simulink model "model_2"  (R2018b)
settings: Solver=VariableStepAuto  StartTime=0.0  StopTime=1  RelTol=1e-6
undefined symbols (not defined in the file): Angle, Magnitude
libraries: powerlib x7, powerlib_meascontrol x2
CloseFcn:
  | location = 0;
  | fault = 1000;
  | volt_mag = Vm(:,2:4);
  | volt_phase = Vp(:,2:4);
  | curr_mag = Im(:,2:4);
  | curr_phase = Ip(:,2:4);
  | logg = [volt_mag,volt_phase,curr_mag,curr_phase];
  | data = xlsread('fdata');
  | data = [data,logg];
  | xlswrite('fdata',data);
settings Model: Creator=Edagotti Pavankumar  LastModifiedBy=Edagotti Pavankumar
settings SolverCC: ZeroCrossAlgorithm=Adaptive
settings DebuggingCC: IgnoredZcDiagnostic=none

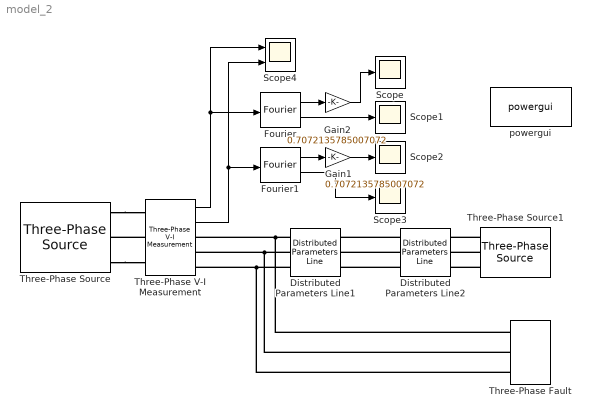
== system model_2 ==
  Distributed Parameters Line1 : powerlib/Elements/Distributed Parameters Line  Phases=3  Frequency=50  Resistance=[0.0238 0.3885]  Inductance="[9.5095e-4  3.25089e-3]"  Capacitance=[12.74e-9 7.751e-9]  Length=180  x1=[8.48515176744739e-11 220461.22116644 220461.22116644;314.159265358979 314.159265358979 314.159265358979;1.82735701330617 0.32640586240689 -1.24439046438801]  x2=[9.7617214960328e-11 220937.914601075 220937.914601075;314.159265358979 314.159265358979 314.159265358979;-2.31830274955501 0.326237122162251 -1.24455920463265]  x3=[1.11025186173268e-12 802.312186393221 802.312186393221;314.159265358979 314.159265358979 314.159265358979;3.10271250295735 0.216627142271568 -1.35416918452333]  x4=[9.65269565360141e-13 802.283126585131 802.283126585132;314.159265358979 314.159265358979 314.159265358979;-0.809925232756074 0.238414402370631 -1.33238192442426]  x5=0.00090355066699992  V1=[8.485e-11 2.205e+05 2.205e+05;314.2 314.2 314.2;1.827 0.3264 -1.244]  V2=[9.762e-11 2.209e+05 2.209e+05;314.2 314.2 314.2;-2.318 0.3262 -1.245]  I1=[1.11e-12 802.3 802.3;314.2 314.2 314.2;3.103 0.2166 -1.354]  I2=[9.653e-13 802.3 802.3;314.2 314.2 314.2;-0.8099 0.2384 -1.332]  nHarmo=1  Measurements=None
      settings: SourceProductName=Simscape Power Systems
  Distributed Parameters Line2 : powerlib/Elements/Distributed Parameters Line  Phases=3  Frequency=50  Resistance=[0.0238 0.3885]  Inductance="[9.5095e-4  3.25089e-3]"  Capacitance=[12.74e-9 7.751e-9]  Length=20  x1=[9.7617214960328e-11 220937.914601075 220937.914601075;314.159265358979 314.159265358979 314.159265358979;-2.06598380399118 0.501194963128134 -1.06960136366676]  x2=[7.31224690470909e-11 220461.378018612 220461.378018612;314.159265358979 314.159265358979 314.159265358979;1.43958780610826 0.50136822766239 -1.06942809913251]  x3=[1.14752079646779e-11 810.765041180401 810.765041180394;314.159265358979 314.159265358979 314.159265358979;-0.0610879160973727 0.588705873026849 -0.982090453768037]  x4=[2.68747980507289e-12 810.674115725578 810.674115725588;314.159265358979 314.159265358979 314.159265358979;-2.96130497430385 0.391966806258209 -1.1788295205367]  x5=0.000100394518555547  V1=[9.762e-11 2.209e+05 2.209e+05;314.2 314.2 314.2;-2.066 0.5012 -1.07]  V2=[7.312e-11 2.205e+05 2.205e+05;314.2 314.2 314.2;1.44 0.5014 -1.069]  I1=[1.148e-11 810.8 810.8;314.2 314.2 314.2;-0.06109 0.5887 -0.9821]  I2=[2.687e-12 810.7 810.7;314.2 314.2 314.2;-2.961 0.392 -1.179]  nHarmo=1  Measurements=None
      settings: SourceProductName=Simscape Power Systems
  Fourier : powerlib_meascontrol/Measurements/Fourier  Freq=50  n=1  InInit=[0, 0]  Ts=0
      settings: SourceProductName=Simscape Power Systems
  Fourier1 : powerlib_meascontrol/Measurements/Fourier  Freq=50  n=1  InInit=[0, 0]  Ts=0
      settings: SourceProductName=Simscape Power Systems
  Gain1 : Gain  Gain=0.7072135785007072
  Gain2 : Gain  Gain=0.7072135785007072
  Scope{,1..3} (4 alike) : Scope
  Scope4 : Scope  NumInputPorts=2
  Three-Phase V-I Measurement : powerlib/Measurements/Three-Phase V-I Measurement  VoltageMeasurement=phase-to-ground  SetLabelV=off  LabelV=Vabc  Vpu=on  VpuLL=off  CurrentMeasurement=yes  SetLabelI=off  LabelI=Iabc  Ipu=on  Pbase=100e6  Vbase=220e3  OutputType=Magnitude-Angle  PhasorSimulation=off  PSBequivalent=0
  Three-Phase Fault : powerlib/Elements/Three-Phase Fault  InitialStates=0  FaultA=off  FaultB=on  FaultC=on  GroundFault=on  SwitchTimes=0.5  External=off  SwitchStatus=NaN  FaultResistance=10  GroundResistance=0.001  SnubberResistance=1e6  SnubberCapacitance=inf  Measurements=None
  Three-Phase Source : powerlib/Electrical Sources/Three-Phase Source  InternalConnection=Yg  VoltagePhases=off  Voltage=220e3  PhaseAngle=0  Voltage_phases=[25e3 25e3 25e3]/sqrt(3)  PhaseAngles_phases=[0 -120 +120]  Frequency=50  NonIdealSource=on  SpecifyImpedance=off  Resistance=0.8929  Inductance=16.58e-3  ShortCircuitLevel=170e6  BaseVoltage=220e3  XRratio=7  BusType=swing  Pref=10e3  Qref=0  Prefabc=[10e3, 10e3, 10e3]  Qrefabc=[0, 0, 0]  Qmin=-inf  Qmax=inf
  Three-Phase Source1 : powerlib/Electrical Sources/Three-Phase Source  InternalConnection=Yg  VoltagePhases=off  Voltage=220e3  PhaseAngle=0  Voltage_phases=[25e3 25e3 25e3]/sqrt(3)  PhaseAngles_phases=[0 -120 +120]  Frequency=50  NonIdealSource=on  SpecifyImpedance=off  Resistance=0.8929  Inductance=16.58e-3  ShortCircuitLevel=176e6  BaseVoltage=220e3  XRratio=7  BusType=swing  Pref=inf  Qref=inf  Prefabc=[10e3, 10e3, 10e3]  Qrefabc=[0, 0, 0]  Qmin=-inf  Qmax=inf
  powergui : powerlib/powergui  Priority=1  SimulationMode=Continuous  SampleTime=50e-10  frequency=50  Iterations=50  frequencyindice=50  Pbase=100e6  ErrMax=1e-4  UnitsV=kV  UnitsW=MW  buscounter=0  FunctionMessages=off  echomessages=off  EnableUseOfTLC=off  CurrentSourceSwitches=off  DisableSnubberDevices=off  DisableRonSwitches=off  DisableVfSwitches=off  DisplayEquations=off  SolverType=Tustin/Backward Euler (TBE)  Interpol=off  ExternalGateDelay=off  methode=off  Ts=100  x0status=blocks  SPID=off  SwTol=0  HookPort=off  RestoreLinks=warning  ResistiveCurrentMeasurement=off  Frange=[0:2:500]  Ylog=off  Xlog=on  ShowGrid=off  save=off  variable=ZData  structure=0  ZoomFFT=off  StartTime=0.0  cycles=1  DisplayStyle=1  fundamental=60  FreqAxis=off  MaxFrequency=1000  frequencyindicesteady=1  RmsSteady=2  display=off
  wires:
  Three-Phase V-I Measurement/1 -> Scope4/1, Fourier/1
  Fourier1/2 -> Scope3/1
  Three-Phase V-I Measurement/2 -> Scope4/2, Fourier1/1
  Fourier/2 -> Scope1/1
  Gain1/1 -> Scope2/1
  Fourier1/1 -> Gain1/1
  Gain2/1 -> Scope/1
  Fourier/1 -> Gain2/1
  connections:
  Three-Phase V-I Measurement/LConn2 -- Three-Phase Source/RConn2
  Three-Phase Source/RConn1 -- Three-Phase V-I Measurement/LConn1
  Three-Phase Source/RConn3 -- Three-Phase V-I Measurement/LConn3
  Distributed Parameters Line1/LConn1 -- Three-Phase Fault/LConn1 -- Three-Phase V-I Measurement/RConn1
  Distributed Parameters Line1/LConn2 -- Three-Phase Fault/LConn2 -- Three-Phase V-I Measurement/RConn2
  Distributed Parameters Line1/LConn3 -- Three-Phase Fault/LConn3 -- Three-Phase V-I Measurement/RConn3
  Distributed Parameters Line2/LConn1 -- Distributed Parameters Line1/RConn1
  Distributed Parameters Line2/LConn2 -- Distributed Parameters Line1/RConn2
  Distributed Parameters Line2/LConn3 -- Distributed Parameters Line1/RConn3
  Three-Phase Source1/RConn1 -- Distributed Parameters Line2/RConn1
  Three-Phase Source1/RConn2 -- Distributed Parameters Line2/RConn2
  Three-Phase Source1/RConn3 -- Distributed Parameters Line2/RConn3
